simulink model "sim_pi_model"  (R2024a)
settings: Solver=ode4  StartTime=0.0  StopTime=1000.0  FixedStep=0.02  RelTol=1e-3
undefined symbols (not defined in the file or in its folder): Ki, Kp, p, r_ref, t_ref
settings Model: Creator=marius  LastModifiedBy=marius

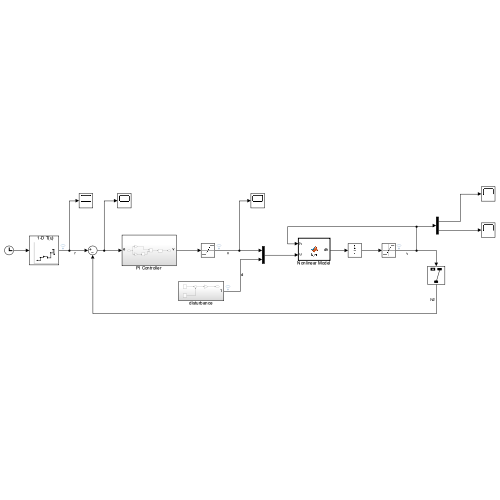
[thumbnail: Simulink's stored preview of the top-level diagram]
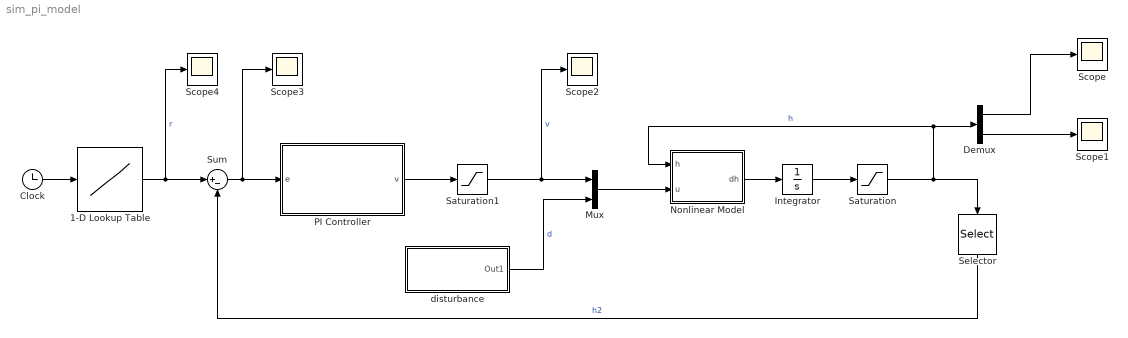
== system sim_pi_model ==
  1-D Lookup Table : Lookup_n-D  NumberOfTableDimensions=1  BreakpointsForDimension1=t_ref  Table=r_ref  InterpMethod=Flat  InternalRulePriority=Speed  RndMeth=Simplest
  Clock : Clock
  Demux : Demux  Outputs=2
  Integrator : Integrator  InitialCondition=[p.h1_bar; p.h2_bar]
  Mux : Mux  Inputs=2
  Nonlinear Model : MATLAB Function  TreatAsAtomicUnit=on
  PI Controller : Subsystem
  Saturation : Saturate  UpperLimit=0.3  LowerLimit=0
  Saturation1 : Saturate  UpperLimit=2*p.v_bar  LowerLimit=0
  Scope{,1..4} (5 alike) : Scope
  Selector : Selector  InputPortWidth=2  IndexOptions=Index vector (dialog)  Indices=2  OutputSizes=1
  Sum : Sum  Inputs=|+-
  disturbance : Subsystem
  wires:
  Nonlinear Model/1(dh) -> Integrator/1
  Integrator/1 -> Saturation/1
  Mux/1 -> Nonlinear Model/2(u)
  PI Controller/1(v) -> Saturation1/1
  Sum/1 -> Scope3/1, PI Controller/1(e)
  Selector/1 -> Sum/2  "h2"
  disturbance/1(Out1) -> Mux/2  "d"
  Demux/1 -> Scope/1
  Demux/2 -> Scope1/1
  Saturation/1 -> Selector/1, Nonlinear Model/1(h), Demux/1  "h"
  Saturation1/1 -> Scope2/1, Mux/1  "v"
  Clock/1 -> 1-D Lookup Table/1
  1-D Lookup Table/1 -> Scope4/1, Sum/1  "r"

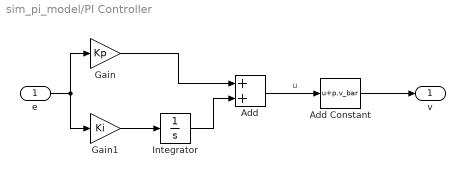
== system sim_pi_model/PI Controller ==
  e : Inport
  Add : Sum
  Add Constant : Bias  Bias=p.v_bar  SaturateOnIntegerOverflow=off
  Gain : Gain  Gain=Kp
  Gain1 : Gain  Gain=Ki
  Integrator : Integrator
  v : Outport
  wires:
  e/1 -> Gain1/1, Gain/1
  Gain1/1 -> Integrator/1
  Integrator/1 -> Add/2
  Gain/1 -> Add/1
  Add/1 -> Add Constant/1  "u"
  Add Constant/1 -> v/1

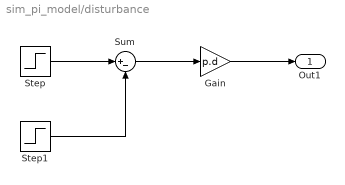
== system sim_pi_model/disturbance ==
  Gain : Gain  Gain=p.d
  Step : Step  Time=p.dt_on  SampleTime=0
  Step1 : Step  Time=p.dt_off  SampleTime=0
  Sum : Sum  Inputs=|+-
  Out1 : Outport
  wires:
  Step/1 -> Sum/1
  Sum/1 -> Gain/1
  Step1/1 -> Sum/2
  Gain/1 -> Out1/1

== matlab function sim_pi_model/Nonlinear Model ==
  data: h input; u input; dh output; p parameter
function dh = fcn(h, u, p)
    [dh, y] = nonlinear_model(h, u, p);
end
